simulink model "TD3_Ex_sim_part1"  (R2022a)
settings: Solver=VariableStepAuto  StartTime=0.0  StopTime=10.0  RelTol=1e-3
undefined symbols (not defined in the file): A, B, C
settings Model: Creator=CS  LastModifiedBy=CS

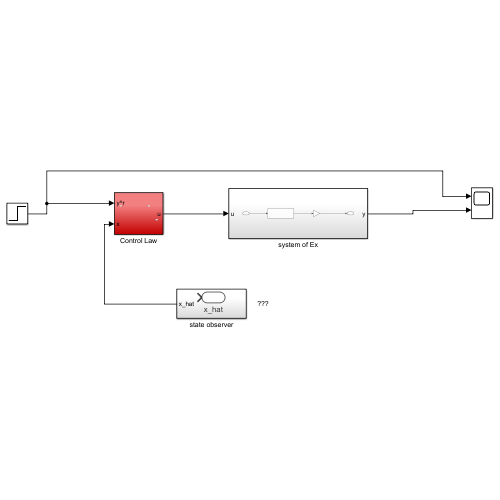
[thumbnail: Simulink's stored preview of the top-level diagram]
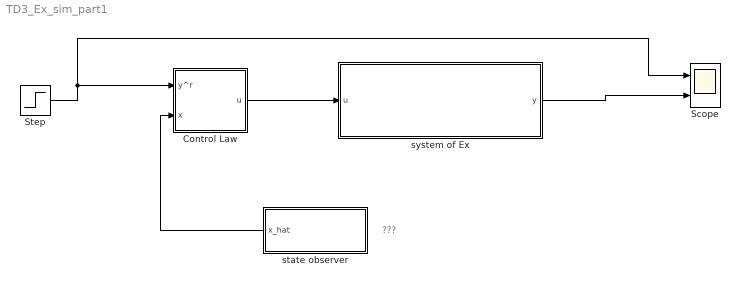
== system TD3_Ex_sim_part1 ==
  note: ???
  Control Law : Subsystem
  Scope : Scope  NumInputPorts=2
  Step : Step  Time=5  SampleTime=0
  state observer : Subsystem
  system of Ex : Subsystem
  wires:
  system of Ex/1(y) -> Scope/2
  Step/1 -> Control Law/1(y^r), Scope/1
  Control Law/1(u) -> system of Ex/1(u)
  state observer/1(x_hat) -> Control Law/2(x)

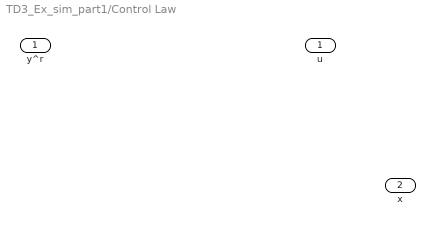
== system TD3_Ex_sim_part1/Control Law ==
  y^r : Inport
  x : Inport  Port=2
  u : Outport

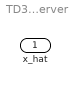
== system TD3_Ex_sim_part1/state observer ==
  x_hat : Outport

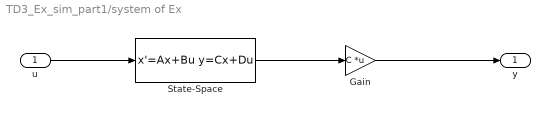
== system TD3_Ex_sim_part1/system of Ex ==
  u : Inport
  Gain : Gain  Gain=C  Multiplication=Matrix(K*u) (u vector)
  State-Space : StateSpace  A=A  B=B  C=eye(3)  D=zeros(3,1)  InitialCondition=0
  y : Outport
  wires:
  u/1 -> State-Space/1
  State-Space/1 -> Gain/1
  Gain/1 -> y/1
